simulink model "DCMG_Kalman_Filter"  (R2024b)
settings: Solver=ode3  StartTime=0.0  StopTime=2  FixedStep=5e-06  RelTol=1e-3
libraries: simulink x3
settings Model: Creator=HP  LastModifiedBy=HP

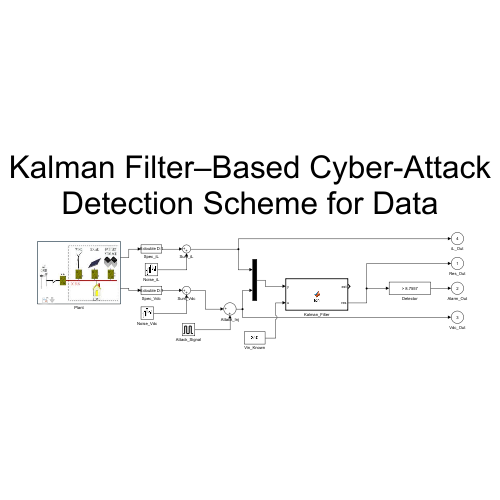
[thumbnail: Simulink's stored preview of the top-level diagram]
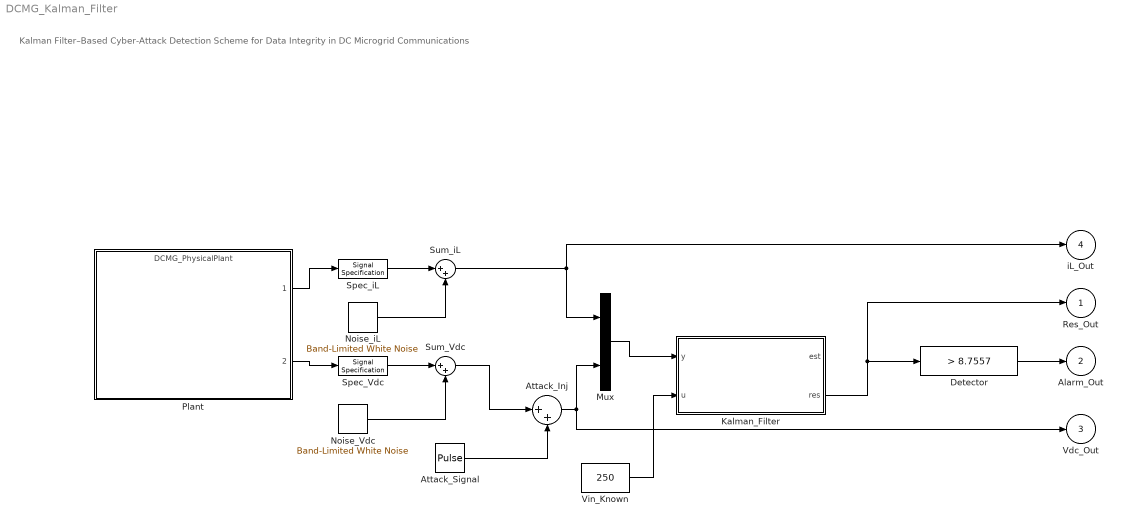
== system DCMG_Kalman_Filter ==
  note: Kalman Filter–Based Cyber-Attack Detection Scheme for Data Integrity in DC Microgrid Communications
  Attack_Inj : Sum  Inputs=|++
  Attack_Signal : DiscretePulseGenerator  PulseType=Time based  Amplitude=20  Period=0.4  PulseWidth=50  PhaseDelay=1.0
  Detector : simulink/Logic and Bit Operations/Compare To Constant  relop=>  const=8.7557  OutDataTypeStr=boolean
  Kalman_Filter : MATLAB Function  TreatAsAtomicUnit=on
  Mux : Mux  Inputs=2
  Noise_Vdc : simulink/Sources/Band-Limited White Noise  Cov=1.25e-06  Ts=5e-06  seed=9981
  Noise_iL : simulink/Sources/Band-Limited White Noise  Cov=1.25e-08  Ts=5e-06  seed=23341
  Plant : ModelReference  ModelNameDialog=DCMG_PhysicalPlant  SimulationMode=Normal  ModelReferenceVersion=14.9
      mask Display: image('download.jpg');
  Spec_Vdc : SignalSpecification  OutDataTypeStr=double  Dimensions=1
  Spec_iL : SignalSpecification  OutDataTypeStr=double  Dimensions=1
  Sum_Vdc : Sum  Inputs=|++
  Sum_iL : Sum  Inputs=|++
  Vin_Known : Constant  Value=250
  Res_Out : Outport
  Alarm_Out : Outport  Port=2
  Vdc_Out : Outport  Port=3
  iL_Out : Outport  Port=4
  wires:
  Plant/1 -> Spec_iL/1
  Plant/2 -> Spec_Vdc/1
  Spec_iL/1 -> Sum_iL/1
  Noise_iL/1 -> Sum_iL/2
  Spec_Vdc/1 -> Sum_Vdc/1
  Noise_Vdc/1 -> Sum_Vdc/2
  Sum_iL/1 -> Mux/1, iL_Out/1
  Sum_Vdc/1 -> Attack_Inj/1
  Attack_Signal/1 -> Attack_Inj/2
  Attack_Inj/1 -> Mux/2, Vdc_Out/1
  Mux/1 -> Kalman_Filter/1(y)
  Vin_Known/1 -> Kalman_Filter/2(u)
  Kalman_Filter/2(res) -> Detector/1, Res_Out/1
  Detector/1 -> Alarm_Out/1

== matlab function DCMG_Kalman_Filter/Kalman_Filter ==
  settings: updateMethod=DISCRETE  sampleTime=5e-06
  data: y input size=[2 1]; u input size=[1 1]; est output size=[2 1]; res output size=[1 1]
function [est, res] = fcn(y, u)
    persistent x_est P Ad Bd Cd Q Rcov
    % Parameters (Imperfect Knowledge)
    Mismatch = 1.1;
    L = 1.8e-3 * Mismatch;
    C = 2.2e-3 / Mismatch;
    R = 6.25; rL = 0.1; Ts = 5e-6;
    % Matrices
    Ac = [-rL/L, -1/L; 1/C, -1/(R*C)];
    Bc = [1/L; 0];
    % Init
    if isempty(x_est)
        Ad = eye(2) + Ac*Ts + (Ac^2 * Ts^2)/2;
        Bd = (eye(2)*Ts + (Ac*Ts^2)/2) * Bc;
        Cd = eye(2);
        x_est = [0; 250];
        P = eye(2);
        Q = eye(2)*1e-5;
        Rcov = eye(2)*0.5;
    end
    % Update
    x_pred = Ad*x_est + Bd*u;
    P_pred = Ad*P*Ad' + Q;
    K = P_pred*Cd'/(Cd*P_pred*Cd' + Rcov);
    x_est = x_pred + K*(y - Cd*x_pred);
    P = (eye(2)-K*Cd)*P_pred;
    est = x_est;
    res = norm(y - Cd*x_pred);
end
